simulink model "P_G_A"  (R2013a)
settings: Solver=ode45  StartTime=0.0  StopTime=0.2  RelTol=1e-3
settings Model: Creator=MEHEDI HASSAN  LastModifiedBy=MEHEDI HASSAN
settings OptimizationCC: InlineParams=on
settings DebuggingCC: SolverPrmCheckMsg=none  ModelReferenceExtraNoncontSigs=none
settings ModelReferenceCC: ModelReferenceNumInstancesAllowed=Single

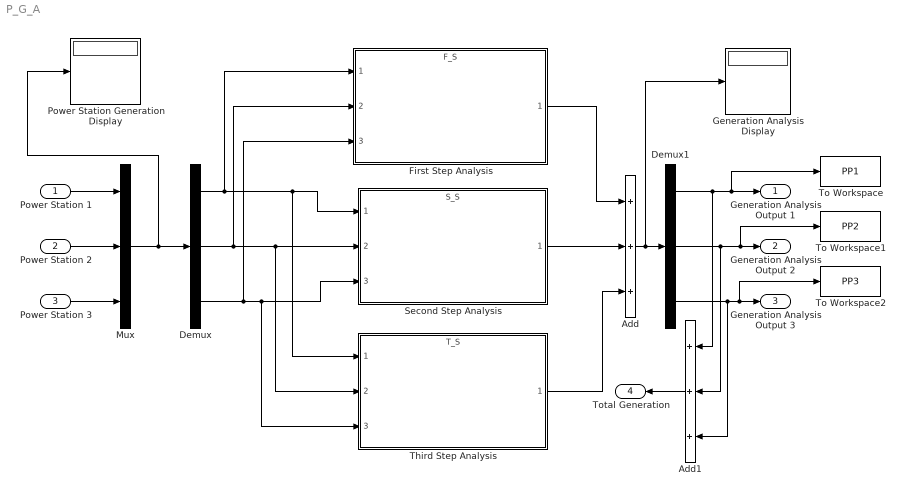
== system P_G_A ==
  Power Station 1 : Inport
  Power Station 2 : Inport  Port=2
  Power Station 3 : Inport  Port=3
  Add : Sum  Inputs=+++
  Add1 : Sum  Inputs=+++
  Demux : Demux  Outputs=3
  Demux1 : Demux  Outputs=3
  First Step Analysis : ModelReference  ModelNameDialog=F_S.slx  SimulationMode=Normal  ModelReferenceVersion=1.15  CopyOfModelName=F_S.slx  DefaultDataLogging=on
  Generation Analysis Display : Display
  Mux : Mux  Inputs=3
  Power Station Generation Display : Display
  Second Step Analysis : ModelReference  ModelNameDialog=S_S.slx  SimulationMode=Normal  ModelReferenceVersion=1.13  CopyOfModelName=S_S.slx  DefaultDataLogging=on
  Third Step Analysis : ModelReference  ModelNameDialog=T_S.slx  SimulationMode=Normal  ModelReferenceVersion=1.13  CopyOfModelName=T_S.slx  DefaultDataLogging=on
  To Workspace : ToWorkspace  VariableName=PP1  SampleTime=-1
  To Workspace1 : ToWorkspace  VariableName=PP2  SampleTime=-1
  To Workspace2 : ToWorkspace  VariableName=PP3  SampleTime=-1
  Generation Analysis Output 1 : Outport
  Generation Analysis Output 2 : Outport  Port=2
  Generation Analysis Output 3 : Outport  Port=3
  "Total Generation " : Outport  Port=4
  wires:
  Mux/1 -> Power Station Generation Display/1, Demux/1
  Demux/2 -> First Step Analysis/2, Second Step Analysis/2, Third Step Analysis/2
  Demux/1 -> First Step Analysis/1, Second Step Analysis/1, Third Step Analysis/1
  Demux/3 -> First Step Analysis/3, Second Step Analysis/3, Third Step Analysis/3
  First Step Analysis/1 -> Add/1
  Second Step Analysis/1 -> Add/2
  Third Step Analysis/1 -> Add/3
  Add/1 -> Demux1/1, Generation Analysis Display/1
  Power Station 1/1 -> Mux/1
  Power Station 2/1 -> Mux/2
  Power Station 3/1 -> Mux/3
  Add1/1 -> "Total Generation "/1
  Demux1/1 -> Add1/1, To Workspace/1, Generation Analysis Output 1/1
  Demux1/2 -> Add1/2, To Workspace1/1, Generation Analysis Output 2/1
  Demux1/3 -> To Workspace2/1, Generation Analysis Output 3/1, Add1/3
